simulink model "aeroblk_calibrated"  (Simulink 6.0)
settings: Solver=FixedStepDiscrete  StartTime=0.0  StopTime=10.0  RelTol=1e-3
PreLoadFcn:
  | aeroblk_aircaldata
values from neighbouring files (symbols this model uses):
  flaps0IAS = 40:10:140    [aeroblk_aircaldata.m]
  flaps10n40IAS = [40:10:80 85]    [aeroblk_aircaldata.m]
libraries: simulink x3, aerolibatmos2 x1, aerolibasang x1
CloseFcn:
  | clear flaps0CAS flaps0IAS flaps10CAS flaps40CAS flaps10n40IAS
settings Model: Creator=The MathWorks Inc.  LastModifiedBy=batserve  ExtModeAutoUpdateStatusClock=off
settings DataIOCC: SaveOutput=off  SaveTime=off  SignalLoggingName=sigsOut
settings OptimizationCC: InlineParams=on
settings DebuggingCC: CheckExecutionContextPreStartOutputMsg=on  CheckExecutionContextRuntimeOutputMsg=on  SolverPrmCheckMsg=none
settings HardwareCC: TargetUnknown=on
settings RTWCC: GenCodeOnly=on

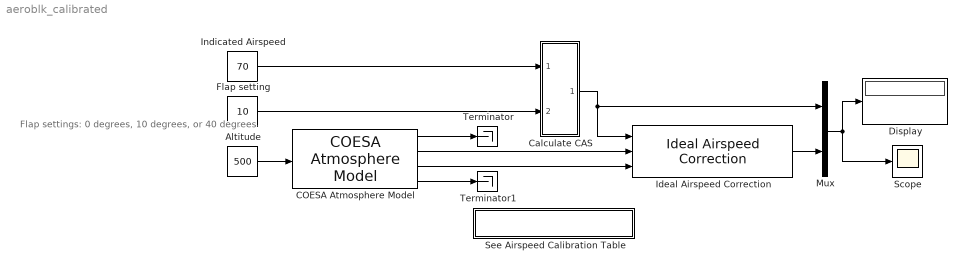
== system aeroblk_calibrated ==
  note: Flap settings:
      |   0 degrees,
      | 10 degrees, or
      | 40 degrees
  Altitude : Constant  Value=500
  COESA Atmosphere Model : aerolibatmos2/COESA Atmosphere Model  units=English (Velocity in kts)  spec=1976 COESA-extended U.S. Standard Atmosphere  model=Profile  profile_var=High temperature  profile_percent=1%  profile_alt=5 km (16404 ft)  envelope_var=High temperature  envelope_percent=1%  action=Warning
  Calculate CAS : Subsystem  PropExecContextAcrossSSBoundary=on
  Display : Display
  Flap setting : Constant  Value=10
  Ideal Airspeed Correction : aerolibasang/Ideal Airspeed Correction  units=English (Velocity in kts)  vel_in=CAS  vel_out_tas=CAS  vel_out_eas=TAS  vel_out_cas=TAS  action=Error
  Indicated Airspeed : Constant  Value=70
  Mux : Mux  Inputs=2
  Scope : Scope
      settings: TimeRange=10  YMin=60  YMax=120
  See Airspeed Calibration Table : Subsystem  PropExecContextAcrossSSBoundary=on
      settings: OpenFcn=open('aeroblk_aircaldata.m');
      mask Display: disp('Cessna 150M Commuter');
  Terminator : Terminator
  Terminator1 : Terminator
  wires:
  COESA Atmosphere Model/3 -> Ideal Airspeed Correction/3
  COESA Atmosphere Model/2 -> Ideal Airspeed Correction/2
  COESA Atmosphere Model/4 -> Terminator1/1
  COESA Atmosphere Model/1 -> Terminator/1
  Altitude/1 -> COESA Atmosphere Model/1
  Flap setting/1 -> Calculate CAS/2(Flap)
  Ideal Airspeed Correction/1 -> Mux/2
  Mux/1 -> Display/1, Scope/1
  Indicated Airspeed/1 -> Calculate CAS/1(IAS)
  Calculate CAS/1(CAS) -> Ideal Airspeed Correction/1, Mux/1

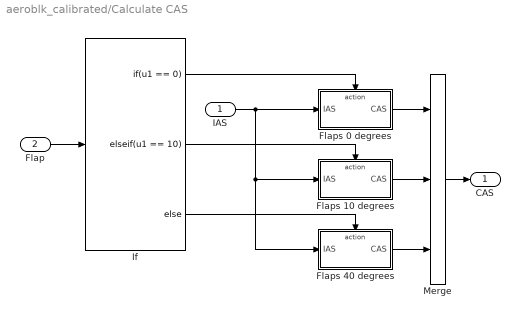
== system aeroblk_calibrated/Calculate CAS ==
  IAS : Inport  Port=1  LatchInput=off
  Flap : Inport  Port=2  LatchInput=off
  Flaps 0 degrees : Subsystem  TreatAsAtomicUnit=on  PropExecContextAcrossSSBoundary=on
  Flaps 10 degrees : Subsystem  TreatAsAtomicUnit=on  PropExecContextAcrossSSBoundary=on
  Flaps 40 degrees : Subsystem  TreatAsAtomicUnit=on  PropExecContextAcrossSSBoundary=on
  If : If  IfExpression=u1 == 0  ElseIfExpressions=u1 == 10
  Merge : Merge  Inputs=3
  CAS : Outport
  wires:
  If/1 -> Flaps 0 degrees/Action
  If/2 -> Flaps 10 degrees/Action
  If/3 -> Flaps 40 degrees/Action
  IAS/1 -> Flaps 0 degrees/1(IAS), Flaps 10 degrees/1(IAS), Flaps 40 degrees/1(IAS)
  Flaps 0 degrees/1(CAS) -> Merge/1
  Flap/1 -> If/1
  Flaps 10 degrees/1(CAS) -> Merge/2
  Flaps 40 degrees/1(CAS) -> Merge/3
  Merge/1 -> CAS/1

== system aeroblk_calibrated/See Airspeed Calibration Table ==

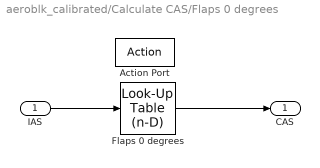
== system aeroblk_calibrated/Calculate CAS/Flaps 0 degrees ==
  IAS : Inport  Port=1  LatchInput=off
  Action Port : ActionPort  ActionType=then
  Flaps 0 degrees : simulink/Look-Up Tables/Look-Up Table (n-D)  numDimsPopupSelect=1  bp1=flaps0IAS  bp2=[10,22,31]  bp3=[1:3]  bp4=[1:3]  bpcell={ [1:3], [1:3] }  explicitNumDims=2  searchMode=Binary Search  cacheBpFlag=off  vectorInputFlag=off  tableData=flaps0CAS  interpMethod=Linear  extrapMethod=None - Clip  rangeErrorMode=Warning
  CAS : Outport
  wires:
  IAS/1 -> Flaps 0 degrees/1
  Flaps 0 degrees/1 -> CAS/1

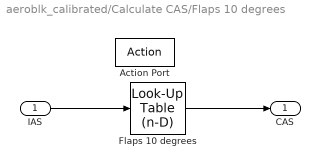
== system aeroblk_calibrated/Calculate CAS/Flaps 10 degrees ==
  IAS : Inport  Port=1  LatchInput=off
  Action Port : ActionPort  ActionType=elseif
  Flaps 10 degrees : simulink/Look-Up Tables/Look-Up Table (n-D)  numDimsPopupSelect=1  bp1=flaps10n40IAS  bp2=[10,22,31]  bp3=[1:3]  bp4=[1:3]  bpcell={ [1:3], [1:3] }  explicitNumDims=2  searchMode=Binary Search  cacheBpFlag=on  vectorInputFlag=off  tableData=flaps10CAS  interpMethod=Linear  extrapMethod=None - Clip  rangeErrorMode=Warning
  CAS : Outport
  wires:
  IAS/1 -> Flaps 10 degrees/1
  Flaps 10 degrees/1 -> CAS/1

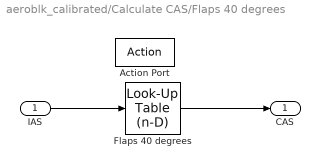
== system aeroblk_calibrated/Calculate CAS/Flaps 40 degrees ==
  IAS : Inport  Port=1  LatchInput=off
  Action Port : ActionPort  ActionType=else
  Flaps 40 degrees : simulink/Look-Up Tables/Look-Up Table (n-D)  numDimsPopupSelect=1  bp1=flaps10n40IAS  bp2=[10,22,31]  bp3=[1:3]  bp4=[1:3]  bpcell={ [1:3], [1:3] }  explicitNumDims=2  searchMode=Binary Search  cacheBpFlag=on  vectorInputFlag=on  tableData=flaps40CAS  interpMethod=Linear  extrapMethod=None - Clip  rangeErrorMode=Warning
  CAS : Outport
  wires:
  IAS/1 -> Flaps 40 degrees/1
  Flaps 40 degrees/1 -> CAS/1
